simulink model "foc_sim"  (R2024b)
settings: Solver=FixedStepDiscrete  StartTime=0.0  StopTime=0.02  FixedStep=Ts  RelTol=1e-3
InitFcn:
  | cd(fileparts(which(bdroot)));
  | foc_params;
undefined symbols (not defined in the file): B, DiscIntNeverNeededParam, iq_ref, J, Ld, Lq, p, Psi_f, Rs, T_load, Ts, V_bus_nom
settings Model: Creator=Administrator  LastModifiedBy=Administrator

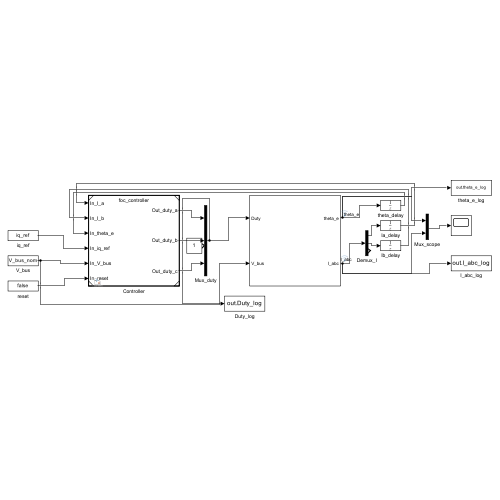
[thumbnail: Simulink's stored preview of the top-level diagram]
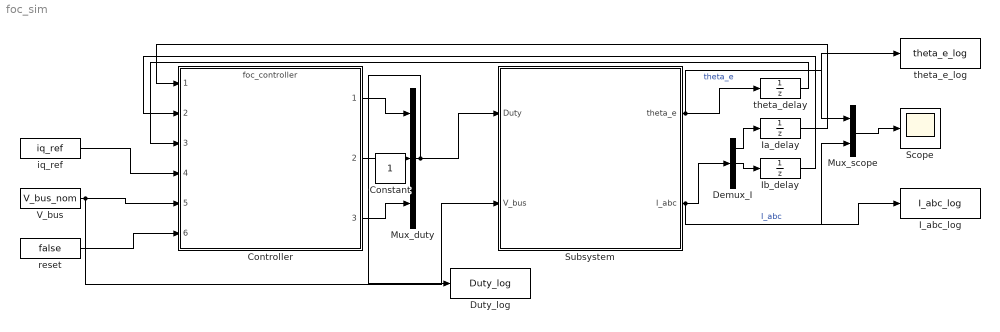
== system foc_sim ==
  Constant : Constant
  Controller : ModelReference  ModelNameDialog=foc_controller  SimulationMode=Normal  ModelReferenceVersion=1.11
  Demux_I : Demux  Outputs=3
  Duty_log : ToWorkspace  VariableName=Duty_log  SaveFormat=Timeseries  SampleTime=-1
  I_abc_log : ToWorkspace  VariableName=I_abc_log  SaveFormat=Timeseries  SampleTime=-1
  Ia_delay : UnitDelay  SampleTime=Ts  HasFrameUpgradeWarning=on
  Ib_delay : UnitDelay  SampleTime=Ts  HasFrameUpgradeWarning=on
  Mux_duty : Mux  Inputs=3
  Mux_scope : Mux  Inputs=2
  Scope : Scope
  Subsystem : Subsystem
  V_bus : Constant  Value=V_bus_nom
  iq_ref : Constant  Value=iq_ref
  reset : Constant  Value=false  OutDataTypeStr=boolean
  theta_delay : UnitDelay  SampleTime=Ts  HasFrameUpgradeWarning=on
  theta_e_log : ToWorkspace  VariableName=theta_e_log  SaveFormat=Timeseries  SampleTime=-1
  wires:
  Controller/1 -> Mux_duty/1
  Controller/2 -> Mux_duty/2
  Controller/3 -> Mux_duty/3
  Mux_duty/1 -> Subsystem/1(Duty), Duty_log/1
  V_bus/1 -> Controller/5, Subsystem/2(V_bus)
  iq_ref/1 -> Controller/4
  Subsystem/2(I_abc) -> Demux_I/1, I_abc_log/1, Mux_scope/2  "I_abc"
  Demux_I/1 -> Ia_delay/1
  Demux_I/2 -> Ib_delay/1
  Ia_delay/1 -> Controller/1
  Ib_delay/1 -> Controller/2
  Subsystem/1(theta_e) -> theta_delay/1, theta_e_log/1, Mux_scope/1  "theta_e"
  theta_delay/1 -> Controller/3
  Mux_scope/1 -> Scope/1
  reset/1 -> Controller/6

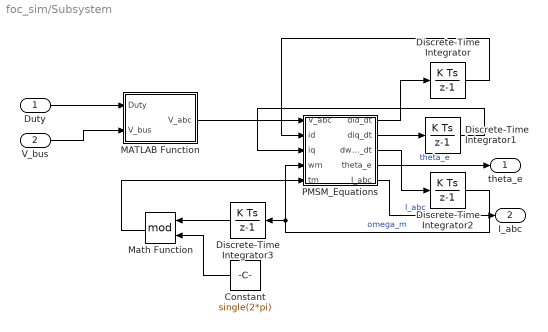
== system foc_sim/Subsystem ==
  Duty : Inport
  V_bus : Inport  Port=2
  Constant : Constant  Value=single(2*pi)  OutDataTypeStr=single
  Discrete-Time Integrator{,1..3} (4 alike) : DiscreteIntegrator  SampleTime=Ts  ICPrevOutput=DiscIntNeverNeededParam  ICPrevScaledInput=DiscIntNeverNeededParam
  MATLAB Function : MATLAB Function  TreatAsAtomicUnit=on
  Math Function : Math  Operator=mod  OutDataTypeStr=single
  PMSM_Equations : MATLAB Function  TreatAsAtomicUnit=on
  theta_e : Outport
  I_abc : Outport  Port=2
  wires:
  Duty/1 -> MATLAB Function/1(Duty)
  V_bus/1 -> MATLAB Function/2(V_bus)
  PMSM_Equations/1(did_dt) -> Discrete-Time Integrator/1
  PMSM_Equations/2(diq_dt) -> Discrete-Time Integrator1/1
  PMSM_Equations/3(dwm_dt) -> Discrete-Time Integrator2/1
  MATLAB Function/1(V_abc) -> PMSM_Equations/1(V_abc)
  Discrete-Time Integrator/1 -> PMSM_Equations/2(id)
  Discrete-Time Integrator1/1 -> PMSM_Equations/3(iq)
  Discrete-Time Integrator2/1 -> PMSM_Equations/4(wm), Discrete-Time Integrator3/1  "omega_m"
  Discrete-Time Integrator3/1 -> Math Function/1
  Constant/1 -> Math Function/2
  Math Function/1 -> PMSM_Equations/5(tm)
  PMSM_Equations/4(theta_e) -> theta_e/1  "theta_e"
  PMSM_Equations/5(I_abc) -> I_abc/1  "I_abc"

== matlab function foc_sim/Subsystem/PMSM_Equations ==
  data: V_abc input size=3; did_dt output single size=1; id input single size=1; iq input single size=1; wm input single size=1; tm input single size=1; diq_dt output single size=1; dwm_dt output single size=1; theta_e output single size=1; I_abc output single size=3; p parameter single; Rs parameter single; Ld parameter single; Lq parameter single; Psi_f parameter single; J parameter single; B parameter single; T_load parameter single
function [did_dt, diq_dt, dwm_dt, theta_e, I_abc] = pmsm_model(V_abc, id, iq, wm, tm, p, Rs, Ld, Lq, Psi_f, J, B, T_load)
    % 1. 机械角转电角度
    theta_e = single(mod(p * tm, 2*pi));
    
    % 2. Clarke & Park 等幅值变换 (V_abc -> V_dq)
    valpha = (2*V_abc(1) - V_abc(2) - V_abc(3)) / 3;
    vbeta  = (sqrt(single(3))*V_abc(2) - sqrt(single(3))*V_abc(3)) / 3;
    vd =  valpha * cos(theta_e) + vbeta * sin(theta_e);
    vq = -valpha * sin(theta_e) + vbeta * cos(theta_e);
    
    % 3. 电流微分计算 (dq轴)
    we = single(p * wm);
    did_dt = (vd - Rs * id + we * Lq * iq) / Ld;
    diq_dt = (vq - Rs * iq - we * Ld * id - we * Psi_f) / Lq;
    
    % 4. 转矩与转速微分计算
    Te = single(1.5) * p * (Psi_f * iq + (Ld - Lq) * id * iq);
    dwm_dt = (Te - T_load - B * wm) / J;
    
    % 5. 反变换输出三相电流 (供外部展示或反馈环测量)
    ialpha = id * cos(theta_e) - iq * sin(theta_e);
    ibeta  = id * sin(theta_e) + iq * cos(theta_e);
    
    ia = ialpha;
    ib = -single(0.5)*ialpha + (sqrt(single(3))/2)*ibeta;
    ic = -single(0.5)*ialpha - (sqrt(single(3))/2)*ibeta;
    I_abc = single([ia; ib; ic]);
end

== matlab function foc_sim/Subsystem/MATLAB Function ==
  data: Duty input size=3; V_abc output size=3; V_bus input size=1
function V_abc = inverter_avg(Duty, V_bus)
    % 桥臂中点相对负极的电压
    v_uo = Duty(1) * V_bus;
    v_vo = Duty(2) * V_bus;
    v_wo = Duty(3) * V_bus;
    
    % 共模中性点电压 (星型接法等效)
    v_n = (v_uo + v_vo + v_wo) / 3;
    
    % 相电压
    v_an = v_uo - v_n;
    v_bn = v_vo - v_n;
    v_cn = v_wo - v_n;
    
    V_abc = single([v_an; v_bn; v_cn]);
end
